simulink library "FIRGenericRmdl"  (R2022b)
settings: Solver=VariableStepAuto  StartTime=0.0  StopTime=10.0  RelTol=1e-3
libraries: FeaturePath x1, ITC x1
settings Model: Creator=ud1041536  LastModifiedBy=kl13806
settings SolverCC: AlgebraicLoopSolver=TrustRegion
settings DebuggingCC: UnconnectedInputMsg=warning  UnconnectedOutputMsg=warning  UnconnectedLineMsg=warning  SFMachineParentedDataDiag=warning  ArithmeticOperatorsInVariantConditions=warning
settings ModelReferenceCC: EnableRefExpFcnMdlSchedulingChecks=on
settings SFSimCC: CustomCodeUndefinedFunction=UseInterfaceOnly
settings RTWCC: DLArmComputeVersion=19.05

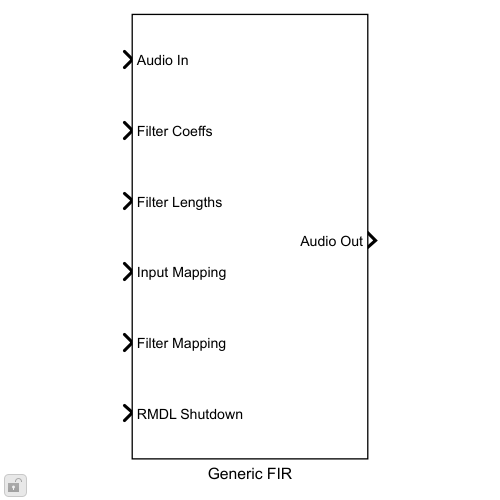
[thumbnail: Simulink's stored preview of the top-level diagram]
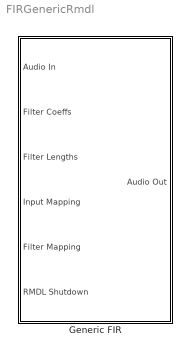
== system FIRGenericRmdl ==
  Generic FIR : Subsystem  mask(FIR Generic){variantSelect=Generic, stateBufferSize=0, numOut=0, frameSize=0, numIn=0}
      mask prompts: variantSelect "Implementation:"; stateBufferSize "State buffer size:"; numOut "Number of outputs:"; frameSize "Frame size:"; numIn "Number of inputs:"
      mask help:
      | Generic FIR is a configurable multi-channel FIR filter that supports one or more channels.  Different filter coefficients and number of coefficients can be used for each channel filter.  There can be fewer inputs than outputs, with some inputs routed to more than one output filter.   Identical filter configurations can also be used for multiple output filters.  The Generic FIR model supports three different implementations, selectable from the model mask:
      |
      | (i)  Core: FIR filters executing on core with target specific CRL support
      | (ii) Accel: FIR filters executing on IIR hardware accelerator, offloading MIPS usage from core
      | (iii) Generic: FIR filters executing on core without CRL support
      |
      | NOTE: The Generic FIR codeWorkMemory buffer should always be mapped to L1 memory or core MIPS usage will increase.
      |
      | For more information, please see 'Help'.
      mask init:
      | % Create alias for code work memory buffer for each instance of model
      | FirGenericMask(gcbh, variantSelect);
      | 
      | % There are three implementation types:
      | % Type    Value  Description
      | % CORE    1      Optimized assembly running on core
      | % ACCEL   2      Computing offloaded to accelerator peripheral
      | % GENERIC 3      Generic implementation for other targets without CRL
      | 
      | if variantSelect == 1
      |     % 6 variable size arrays (for input, coeffs, states, 
      |     % stateSharingEnabled, taps array per output channel,
      |     % and mapped audio input offsets) 
      |     % + 10 struct members
      |     codeWorkMemorySize = numOut * 6 + 10;  % words
      |     
      | elseif variantSelect == 2
      |     % Accelerator CRL code work memory size is equal to:
      |     %             sizeof(accelWorkMemory_t) + variableDataSize;
      |     % with variable data size dependent on number inputs, number outputs
      |     % and frame size.  NOTE: this must be updated to match the CRL code
      |     % if any changes are made to the accelWorkMemory_t structure.
      |     codeWorkMemorySize = 112 + (24 + numIn*48 + numOut*(80 + 4*frameSize));  % bytes
      |     codeWorkMemorySize = codeWorkMemorySize / 4;  % words (single)
      |     
      | else
      |     % This is not used if there is no CRL
      |     codeWorkMemorySize = 1;
      | end
      mask Help:
      | Generic multi-channel FIR block supports multiple inputs, outputs and coefficient sets. Some inputs may drive multiple outputs, and this input sharing is specified by an input mapping per output. Some filters may be shared among multiple outputs, and this filter sharing is specified by a filter mapping per output. Input sharing assumes all filters sharing the same input have the same length to support state buffer sharing.
      | 
      | <b>Input signals: </b>
      | u: input channels [frame size x number of inputs]
      | coeffs: coefficient sets [total sum of filter lengths x 1]
      | filterLengths: array of filter lengths [number of filters x 1]
      | inputMapping: zero-based input mapping for each output [number of outputs x 1]
      | filterMapping:  zero-based filter mapping for each output [number of outputs x 1]
      | RMDLshutdown: shutdown enable to indicate a feature specific RMDL is starting [1 x 1]
      | 
      | <b>Output signals: </b>
      | y: output channels [frame size x number of outputs]
      | 
      | <b>Mask parameters: </b>
      | Implementation: Core/Accel /Generic
      | State buffer size: total size of state buffer [total state buffer size x 1]
      | Number of outputs
      | Frame size
      | Number of inputs
      mask TypeOptions variantSelect: Core | Accel | Generic
      mask Callback variantSelect:
      | % Get the mask parameter value
      | maskStr = get_param(gcb,'variantSelect');
      | 
      | % Check the value of 'variantSelect'
      | if (~strcmp(maskStr,"Accel"))
      |     % Turn the visibility of 'frameSize' and 'numChannels' OFF
      |     set_param(gcb,'MaskVisibilities',{'on';'on';'on';'off';'off'});
      | else
      |     % "Accel": Set the visibility of all parameters to ON
      |     set_param(gcb,'MaskVisibilities',{'on';'on';'on';'on';'on'});
      | end

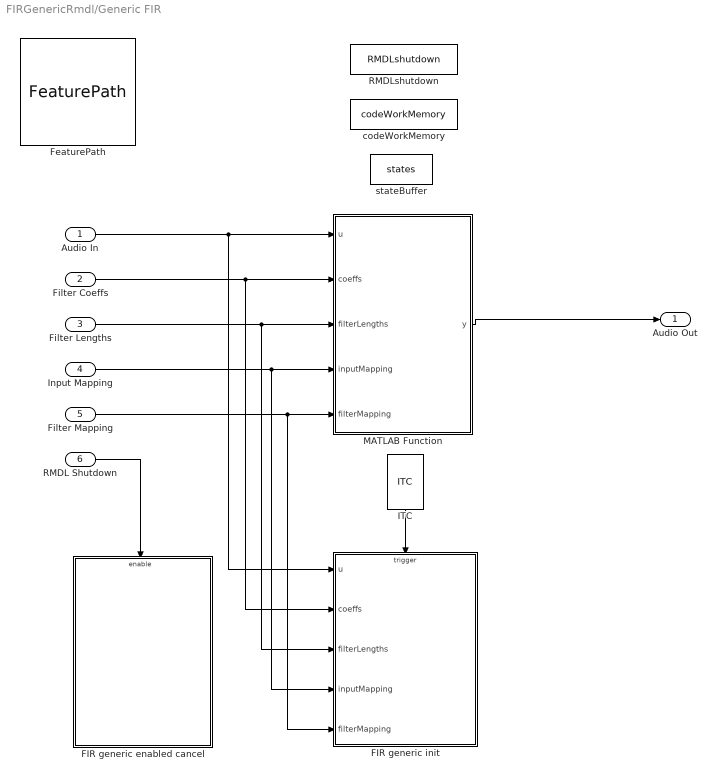
== system FIRGenericRmdl/Generic FIR ==
  Audio In : Inport
  Filter Coeffs : Inport  Port=2
  Filter Lengths : Inport  Port=3
  Input Mapping : Inport  Port=4
  Filter Mapping : Inport  Port=5
  RMDL Shutdown : Inport  Port=6
  FIR generic enabled cancel : Subsystem  TreatAsAtomicUnit=on
  FIR generic init : MATLAB Function  TreatAsAtomicUnit=on  RTWFcnName=foo
  FeaturePath : FeaturePath/FeaturePath  FeatureName=FIR  IsGroup=off  GroupNumber=-1  IsModule=off  TriggerInit=[205 -116 320 -9]
      settings: SourceProductName=Bose Talaria
  ITC : ITC/ITC
      settings: SourceProductName=Bose Talaria
  MATLAB Function : MATLAB Function  TreatAsAtomicUnit=on
  RMDLshutdown : DataStoreMemory  DataStoreName=RMDLshutdown  WriteAfterWriteMsg=warning  ShowAdditionalParam=off  OutDataTypeStr=uint32  Dimensions=[1,1]
      settings: LockScale=on
  codeWorkMemory : DataStoreMemory  DataStoreName=codeWorkMemory  WriteAfterWriteMsg=warning  InitialValue=zeros(1,codeWorkMemorySize)  EmbeddedSignalClassName=Blocklib.Signal  ShowAdditionalParam=off  OutDataTypeStr=uint32
  stateBuffer : DataStoreMemory  DataStoreName=states  ReadBeforeWriteMsg=warning  WriteAfterWriteMsg=warning  WriteAfterReadMsg=warning  InitialValue=zeros(stateBufferSize,1)  EmbeddedSignalClassName=Blocklib.Signal  ShowAdditionalParam=off  OutDataTypeStr=single
  Audio Out : Outport  VectorParamsAs1DForOutWhenUnconnected=off
  wires:
  Filter Lengths/1 -> MATLAB Function/3(filterLengths), FIR generic init/3(filterLengths)
  Input Mapping/1 -> MATLAB Function/4(inputMapping), FIR generic init/4(inputMapping)
  Filter Coeffs/1 -> FIR generic init/2(coeffs), MATLAB Function/2(coeffs)
  Filter Mapping/1 -> MATLAB Function/5(filterMapping), FIR generic init/5(filterMapping)
  MATLAB Function/1(y) -> Audio Out/1
  ITC/1 -> FIR generic init/Trigger
  Audio In/1 -> FIR generic init/1(u), MATLAB Function/1(u)
  RMDL Shutdown/1 -> FIR generic enabled cancel/Enable

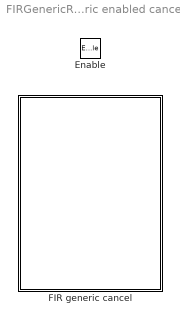
== system FIRGenericRmdl/Generic FIR/FIR generic enabled cancel ==
  Enable : EnablePort
  FIR generic cancel : MATLAB Function  TreatAsAtomicUnit=on

== matlab function FIRGenericRmdl/Generic FIR/FIR generic init ==
  data: u input; coeffs input; filterLengths input; inputMapping input; filterMapping input; states data_store_memory; codeWorkMemory data_store_memory; variantSelect parameter; RMDLshutdown data_store_memory
  events: trigger input FUNCTION_CALL_EVENT
function fir_generic_init(u,coeffs, filterLengths, inputMapping, filterMapping, variantSelect)

% Generic FIR function to work with M inputs, N outputs and K filters
%
% Parameters:
%   u:              input channels [frame size x number of inputs]
%   coeffs:         coefficient sets [total filter lengths x 1]
%   filterLengths:  array of filter lengths [number of filters x 1]
%   inputMapping:   zero-based input mapping for each filter  [number of outputs x 1]
%   filterMapping:  zero-based filter mapping for each filter [number of outputs x 1]
%
% Global parameters:
%   states:         array of states [totalBufferSize x 1]
%   codeWorkMemory: working memory set up during roommode reset/init CRL
%                   function call [codeWorkMemorySize x 1]
%   RMDLshutdown: Flag to indicate RMDL is in progress [1 x 1]

% Extract configuration information from inputs
[frame_size, num_inputs]  = size(u);
num_outputs = numel(inputMapping);

global states;
global codeWorkMemory;
global RMDLshutdown;

% Get the work memory and states size
workMemorySize = numel(codeWorkMemory);
statesSize = numel(states);

% Set correct data types
filter_length = uint32(filterLengths);
numCoeffSets = uint32(numel(filter_length));
frame_size = uint32(frame_size);
num_outputs = uint32(num_outputs);
num_inputs = uint32(num_inputs);
workMemorySize = uint32(workMemorySize);
statesSize = uint32(statesSize);
    
% There are three implementation types:
% Type    Value   Description
% CORE    1       Optimized assembly running on core
% ACCEL   2       Computing offloaded to accelerator peripheral
% GENERIC 3       Generic implementation for other targets without CRL 
%
% NOTE: GENERIC implementation does not use codeWorkMemory, thus does not
% need any custom initialization.
if (variantSelect == 1)
    y = fir_core_init(u, coeffs, states, filter_length, inputMapping, filterMapping, frame_size, numCoeffSets, num_inputs, num_outputs, codeWorkMemory);
    
    % NOTE: The CRL mechanism requires an output for the function call,
    % and appears to be optimized out if that return value isn't used. 
    % This is a dummy operation to make sure CRL ends up in generated code
    codeWorkMemory(1) = y; 
elseif (variantSelect == 2)
    y = fir_accelerator_init(u, coeffs, states, statesSize, filter_length, inputMapping, filterMapping, frame_size, ...
                             numCoeffSets, num_inputs, num_outputs, codeWorkMemory, workMemorySize);
    
    % NOTE: The CRL mechanism requires an output for the function call,
    % and appears to be optimized out if that return value isn't used. 
    % This is a dummy operation to make sure CRL ends up in generated code
    codeWorkMemory(1) = y; 
end

% Set flag to indicate initialization has completed and step functions can
% start running.
RMDLshutdown = uint32(1);

end


function y = fir_accelerator_init(u, coeffs, states, statesSize, filterLengths, inputMapping, filterMapping,...
                                  frameSize, numCoeffSets, numInputs, numOutputs, workMemory,...
                                  workMemorySize)                         
% If target == codegen, error out if no CRL found
coder.replace('-errorifnoreplacement');

% No init simulation code, but need to do something to ensure CRL does not
% get optimized out
y = workMemory(1) + 1;

end

function y = fir_core_init(u, coeffs, states, filterLengths, inputMapping, filterMapping,...
                             frameSize, numCoeffSets, numInputs, numOutputs, workMemory)
% If target == codegen, error out if no CRL found
coder.replace('-errorifnoreplacement');

% No init simulation code, but need to do something to ensure CRL does not
% get optimized out
y = workMemory(1) + 1;

end

== matlab function FIRGenericRmdl/Generic FIR/MATLAB Function ==
  data: u input; y output; coeffs input; filterLengths input; inputMapping input; filterMapping input; states data_store_memory; variantSelect parameter; codeWorkMemory data_store_memory; RMDLshutdown data_store_memory
function y = fir_generic(u, coeffs, filterLengths, inputMapping, filterMapping, variantSelect)
% Generic FIR function to work with M inputs, N outputs and K filters
%
% Parameters:
%   u:              input channels [frame size x number of inputs]
%   coeffs:         coefficient sets [total filter lengths x 1]
%   filterLengths:  array of filter lengths [number of filters x 1]
%   inputMapping:   zero-based input mapping for each filter  [number of outputs x 1]
%   filterMapping:  zero-based filter mapping for each filter [number of outputs x 1]
%
% Global parameters:
%   states:         array of states [totalBufferSize x 1]
%   codeWorkMemory: working memory set up during roommode reset/init CRL
%                   function call [codeWorkMemorySize x 1]
%   RMDLshutdown: Flag to indicate RMDL is in progress [1 x 1]

% Extract configuration information from inputs
[frame_size, num_inputs]  = size(u);
num_outputs = numel(inputMapping);

global states;
global codeWorkMemory;
global RMDLshutdown;

% Do not call the step processing functions if RMDL shutdown is in
% progress
if (RMDLshutdown == 0)
    y = zeros(frame_size, num_outputs, 'single');
    return;
end

% Set correct data types
filter_length = uint32(filterLengths);
frame_size = uint32(frame_size);
num_outputs = uint32(num_outputs);
num_inputs = uint32(num_inputs);

% Define one-frame delay buffer only for Accelerator simulation 
% Simulink will optimize this out for code generation
persistent delayedOut;
if isempty(delayedOut)
    delayedOut = single(zeros(frame_size, num_outputs));
end
    
% There are three implementation types:
% Type    Value   Description
% CORE    1       Optimized assembly running on SHARC+ core
% ACCEL   2       Computing offloaded to SHARC+ accelerator peripheral
% GENERIC 3       Generic implementation for other targets without CRL

% Simulation
if(coder.target('MATLAB') || coder.target('Sfun')) 
    if (variantSelect == 2)
        % Manually insert one-frame delay in simulation to mimic 
        % Accelerator behavior
        y = delayedOut;
        delayedOut = fir_generic_simulation(u, coeffs, states, filter_length, inputMapping, ...
                filterMapping, frame_size, num_inputs, num_outputs);
    else
        y = fir_generic_simulation(u, coeffs, states, filter_length, inputMapping, ...
                filterMapping, frame_size, num_inputs, num_outputs);
    end

% Code generation
else 
    if (variantSelect == 1)
        y = fir_core_process(u, codeWorkMemory, num_outputs);
    elseif (variantSelect == 2)
        y = fir_accelerator_process(u, codeWorkMemory, num_outputs);
    else
        y = fir_generic_simulation(u, coeffs, states, filter_length, inputMapping, ...
                filterMapping, frame_size, num_inputs, num_outputs);
    end  
end

end


%% CRL functions for code generation
function y = fir_core_process(u, workMemory, numOutputs)
% If target == codegen, error out if no CRL found
coder.replace('-errorifnoreplacement');
[frameSize, ~]  = size(u);
y = single(zeros(frameSize, numOutputs));
end

function y = fir_accelerator_process(u, workMemory, numOutputs)
% If target == codegen, error out if no CRL found
coder.replace('-errorifnoreplacement');
[frameSize, ~]  = size(u);
y = single(zeros(frameSize, numOutputs));
end

== matlab function FIRGenericRmdl/Generic FIR/FIR generic enabled cancel/FIR generic cancel ==
  data: variantSelect parameter; codeWorkMemory data_store_memory; RMDLshutdown data_store_memory
function fir_generic_cancel(variantSelect)

% FIR accelerator function stops step/process function from running on each
% frame and cancels FIR accelerator task if currently active.
% 
% Parameters:
%   None
%
% Global parameters:
%   codeWorkMemory: Working memory set up during roommode reset/init CRL
%                   function call [1 x codeWorkMemorySize]
%   RMDLshutdown: Flag to indicate RMDL is in progress [1 x 1] 

global codeWorkMemory;
global RMDLshutdown;

% Clear flag to indicate RMDL shutdown has started. Note that this flag
% will be set after RMDL and initialization have completed.
RMDLshutdown = uint32(0);

% There are three implementation types:
% Type    Value   Description
% CORE    1       Optimized assembly running on core
% ACCEL   2       Computing offloaded to accelerator peripheral
% GENERIC 3       Generic implementation for other targets without CRL 
if(~coder.target('MATLAB') && ~coder.target('Sfun')) 
    % Code Generation
    if (variantSelect == 2)
        y = fir_accelerator_cancel(codeWorkMemory);

        % NOTE: The CRL mechanism requires an output for the function call,
        % and appears to be optimized out if that return value isn't used. 
        % This is a dummy operation to make sure CRL ends up in generated code
        codeWorkMemory(1) = y;
    end
end

end


% FIR accelerator CRL cancel function conceptual specification
function y = fir_accelerator_cancel(workMemory)
% If target == codegen, error out if no CRL found
coder.replace('-errorifnoreplacement');

% No cancel simulation code, but need to do something to ensure CRL does not
% get optimized out
y = uint32(workMemory(1) + 1);

end
